simulink model "TP4_control_adaptivo_mod_completo"  (R2024b)
settings: Solver=VariableStepAuto  StartTime=0.0  StopTime=10.0  FixedStep=0.  RelTol=1e-3
undefined symbols (not defined in the file): mu_est0, states0, v0
settings Model: Creator=tomii  LastModifiedBy=tomii

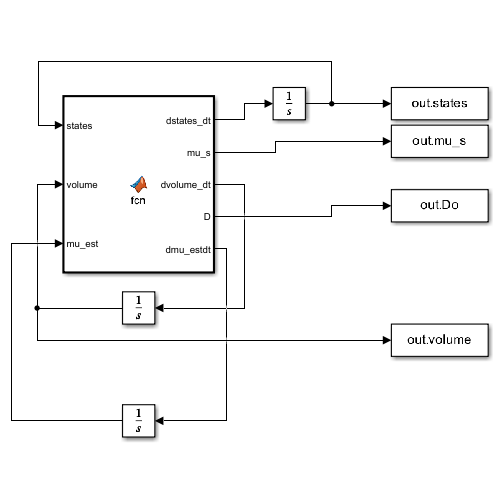
[thumbnail: Simulink's stored preview of the top-level diagram]
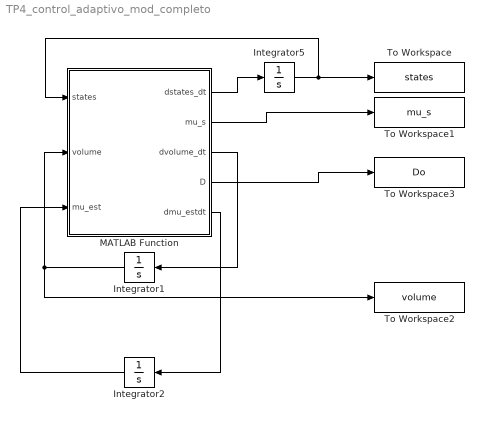
== system TP4_control_adaptivo_mod_completo ==
  Integrator1 : Integrator  InitialCondition=v0
  Integrator2 : Integrator  InitialCondition=mu_est0
  Integrator5 : Integrator  InitialCondition=states0
  MATLAB Function : MATLAB Function  TreatAsAtomicUnit=on
  To Workspace : ToWorkspace  VariableName=states  SaveFormat=Timeseries  SampleTime=-1
  To Workspace1 : ToWorkspace  VariableName=mu_s  SaveFormat=Timeseries  SampleTime=-1
  To Workspace2 : ToWorkspace  VariableName=volume  SaveFormat=Timeseries  SampleTime=-1
  To Workspace3 : ToWorkspace  VariableName=Do  SaveFormat=Timeseries  SampleTime=-1
  wires:
  MATLAB Function/1(dstates_dt) -> Integrator5/1
  Integrator5/1 -> MATLAB Function/1(states), To Workspace/1
  MATLAB Function/2(mu_s) -> To Workspace1/1
  MATLAB Function/3(dvolume_dt) -> Integrator1/1
  Integrator1/1 -> MATLAB Function/2(volume), To Workspace2/1
  MATLAB Function/4(D) -> To Workspace3/1
  Integrator2/1 -> MATLAB Function/3(mu_est)
  MATLAB Function/5(dmu_estdt) -> Integrator2/1

== matlab function TP4_control_adaptivo_mod_completo/MATLAB Function ==
  data: dstates_dt output; mu_s output; states input; volume input; mu_est input; modelParameters parameter; dvolume_dt output; D output; dmu_estdt output
function [dstates_dt, mu_s, dvolume_dt, D, dmu_estdt] = fcn(states, volume, mu_est, modelParameters)   
    
    K=modelParameters.K;
    xi_in=modelParameters.xi_in;
    ks1=modelParameters.ks1;
    gamma1=modelParameters.gamma1;
    
    s_r=modelParameters.s_r;
    s_in=modelParameters.s_in;

    qp_max=modelParameters.qp_model.qp_max;
    Kps=modelParameters.qp_model.Kps;
    Kips=modelParameters.qp_model.Kips;
    Kipn=modelParameters.qp_model.Kipn;

    Kn=modelParameters.mu_model.Kn;
    Ks=modelParameters.mu_model.Ks;
    Kis=modelParameters.mu_model.Kis;
    mu_max=modelParameters.mu_model.mu_max;

    x=states(1);
    s=states(2);
    n=states(3);
    p=states(4);

    qp_s=qp_max*(s/(Kps+s+s*s/Kips))*(Kipn/(Kipn+n));
    mu_s=mu_max*(s/(Ks+s+s*s/Kis))*(n/(Kn+n));
    rx=x*mu_s;
    rp=x*qp_s;

    D=(ks1*x*mu_est+gamma1*(s_r-s))/(s_in-s);
    dmu_estdt = gamma1*(ks1*x)*(s_r-s);

    dstates_dt = K * [rx;rp] + D*(xi_in-states);
    dvolume_dt = 0;

end
